simulink model "c166_user_io"  (Simulink 6.0)
settings: Solver=ode45  StartTime=0.0  StopTime=100  FixedStep=0.01  RelTol=1e-3
PreLoadFcn:
  | RTWConfigurationCB('preloadfcn', bdroot);
  | 
  | 
  | 
  | 
  | c166useriodata
libraries: c166drivers x1
CloseFcn:
  | rtwprivate ssgencode ModelCloseRequest c166_user_io
settings Model: Creator=The MathWorks Inc.  LastModifiedBy=batserve  ExtModeAutoUpdateStatusClock=off  ProdHWDeviceType=Infineon C16x
settings DataIOCC: SaveFormat=Structure  SignalLoggingName=sigsOut
settings OptimizationCC: InlineParams=on  InlineInvariantSignals=off  ZeroExternalMemoryAtStartup=off  ZeroInternalMemoryAtStartup=off  InitFltsAndDblsToZero=off  LifeSpan=1
settings DebuggingCC: CheckExecutionContextPreStartOutputMsg=on  CheckExecutionContextRuntimeOutputMsg=on  SolverPrmCheckMsg=none
settings HardwareCC: ProdBitPerInt=16  ProdEndianess=LittleEndian  ProdWordSize=16  ProdHWDeviceType=Infineon C16x  TargetHWDeviceType=32-bit Generic
settings RTWCC: SystemTargetFile=c166.tlc  MakeCommand=make_rtw_user  TemplateMakefile=c166.tmf  ProcessScript=c166_make_rtw_hook
settings CodeAppCC: IgnoreCustomStorageClasses=off
settings STFCustomTargetCC: TargetFcnLib=ansi_tfl_tmw.mat  GenFloatMathFcnCalls=ANSI_C  GenerateSampleERTMain=on  IncludeMdlTerminateFcn=off  CombineOutputUpdateFcns=on  ERTCustomFileBanners=on  SupportNonFinite=off  SupportComplex=off  PurelyIntegerCode=on  SystemTargetFile=c166.tlc
settings ERTTargetCC: TargetFcnLib=ansi_tfl_tmw.mat  GenFloatMathFcnCalls=ANSI_C  GenerateSampleERTMain=on  IncludeMdlTerminateFcn=off  SupportNonFinite=off  SupportComplex=off  PurelyIntegerCode=on  SupportContinuousTime=on  SupportNonInlinedSFcns=on  RootIOFormat=Individual Arguments  ERTCustomFileTemplate=example_file_process.tlc  InitialValueSource=Model
settings CustomProperty: DataType=RTWOptions_EnumType__toolbox_rtw_targets_c166_c166_c166_BuildActionC166  Value=Download_and_run
settings EnumStrPairs: String=Run_with_simulator

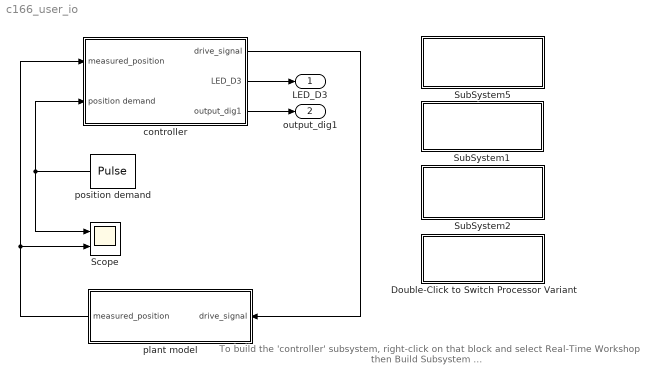
== system c166_user_io ==
  note: To build the 'controller'
      | subsystem, right-click
      | on that block and select
      | Real-Time Workshop
      | then Build Subsystem ...
  Double-Click to Switch Processor Variant : Subsystem  PropExecContextAcrossSSBoundary=on
      settings: OpenFcn=c166switchconfig(gcs)
      mask Display: disp('Switch Target\nProcessor Variant');
  Scope : Scope  NumInputPorts=2
      settings: YMin=0~0  YMax=600~600
  SubSystem1 : Subsystem  PropExecContextAcrossSSBoundary=on
      settings: OpenFcn=edit c166useriodata.m
      mask Display: disp('Open custom storage\nclass data file');
  SubSystem2 : Subsystem  PropExecContextAcrossSSBoundary=on
      settings: OpenFcn=helpview([docroot '/toolbox/c166/c166.map'], 'c166_user_io');
      mask Display: disp('Open help for\nintegrating hand code');
  SubSystem5 : Subsystem  PropExecContextAcrossSSBoundary=on
      settings: OpenFcn=|
      | edit([ matlabroot '/toolbox/rtw/targets/c166/c166demos/user_src/user_io.h'])
      | edit([ matlabroot '/toolbox/rtw/targets/c166/c166demos/user_src/user_io.c'])
      mask Display: disp('Open i/o driver\nsource files');
  controller : Subsystem  InitFcn=|  PropExecContextAcrossSSBoundary=on
      | % START RTW CONFIGURATION CODE %
      | RTWConfigurationCB('rtw_target_initfcn',gcb);
      | % END RTW CONFIGURATION CODE %
      mask Display: image(imread('target_affordance_icon.jpg'),'bottom-right')
  plant model : Subsystem  Orientation=left  PropExecContextAcrossSSBoundary=on
  position demand : DiscretePulseGenerator  Orientation=left  PulseType=Time based  Amplitude=uint16(512)  Period=5  PulseWidth=50
  LED_D3 : Outport
  output_dig1 : Outport  Port=2
  wires:
  controller/2(LED_D3) -> LED_D3/1
  controller/1(drive_signal) -> plant model/1(drive_signal)
  plant model/1(measured_position) -> controller/1(measured_position), Scope/2
  position demand/1 -> controller/2(position demand), Scope/1
  controller/3(output_dig1) -> output_dig1/1

== system c166_user_io/Double-Click to Switch Processor Variant ==

== system c166_user_io/SubSystem1 ==

== system c166_user_io/SubSystem2 ==

== system c166_user_io/SubSystem5 ==

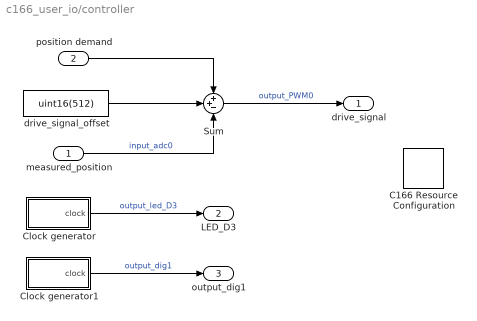
== system c166_user_io/controller ==
  measured_position : Inport  Port=1  SampleTime=0.001  LatchInput=off
  position demand : Inport  Port=2  SampleTime=0.001  LatchInput=off
  C166 Resource Configuration : c166drivers/C166 Resource Configuration  Tag=RTW CONFIGURATION BLOCK  Priority=-100000  oldParentName=c166_user_io/controller  oldBlockName=|  defaultConfigLibrary=c166drivers
      | c166_user_io/controller/C166
      | Resource
      | Configuration
  Clock generator : Subsystem  PropExecContextAcrossSSBoundary=on
  Clock generator1 : Subsystem  PropExecContextAcrossSSBoundary=on
  Sum : Sum  Inputs=++-  OutDataTypeMode=uint16  SaturateOnIntegerOverflow=on
  drive_signal_offset : Constant  Value=uint16(512)
  drive_signal : Outport
  LED_D3 : Outport  Port=2
  output_dig1 : Outport  Port=3
  wires:
  measured_position/1 -> Sum/3  "input_adc0"
  Sum/1 -> drive_signal/1  "output_PWM0"
  Clock generator/1(clock) -> LED_D3/1  "output_led_D3"
  drive_signal_offset/1 -> Sum/2
  position demand/1 -> Sum/1
  Clock generator1/1(clock) -> output_dig1/1  "output_dig1"

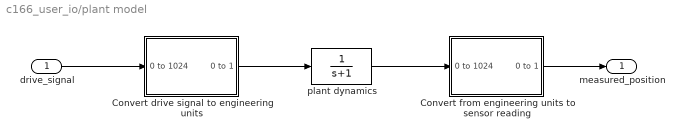
== system c166_user_io/plant model ==
  drive_signal : Inport  Port=1  LatchInput=off
  Convert drive signal to engineering units : Subsystem  PropExecContextAcrossSSBoundary=on
  Convert from engineering units to sensor reading : Subsystem  PropExecContextAcrossSSBoundary=on
  plant dynamics : TransferFcn  Denominator=[1 1]
  measured_position : Outport
  wires:
  drive_signal/1 -> Convert drive signal to engineering units/1(0 to 1024)
  Convert drive signal to engineering units/1(0 to 1) -> plant dynamics/1
  plant dynamics/1 -> Convert from engineering units to sensor reading/1(0 to 1024)
  Convert from engineering units to sensor reading/1(0 to 1) -> measured_position/1

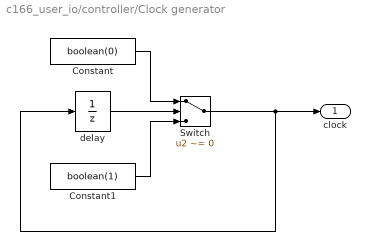
== system c166_user_io/controller/Clock generator ==
  Constant : Constant  Value=boolean(0)
  Constant1 : Constant  Value=boolean(1)
  Switch : Switch  Criteria=u2 ~= 0  SaturateOnIntegerOverflow=on
  delay : UnitDelay  X0=boolean(0)
  clock : Outport
  wires:
  delay/1 -> Switch/2
  Switch/1 -> clock/1, delay/1
  Constant/1 -> Switch/1
  Constant1/1 -> Switch/3

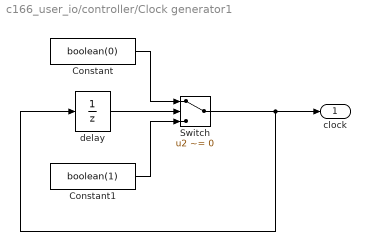
== system c166_user_io/controller/Clock generator1 ==
  Constant : Constant  Value=boolean(0)
  Constant1 : Constant  Value=boolean(1)
  Switch : Switch  Criteria=u2 ~= 0  SaturateOnIntegerOverflow=on
  delay : UnitDelay  X0=boolean(0)
  clock : Outport
  wires:
  Constant1/1 -> Switch/3
  Constant/1 -> Switch/1
  Switch/1 -> delay/1, clock/1
  delay/1 -> Switch/2

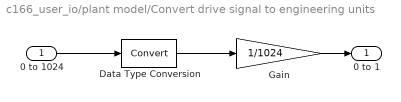
== system c166_user_io/plant model/Convert drive signal to engineering units ==
  0 to 1024 : Inport  Port=1  LatchInput=off
  Data Type Conversion : DataTypeConversion  OutDataTypeMode=double  SaturateOnIntegerOverflow=on  RndMeth=Zero
  Gain : Gain  Gain=1/1024  SaturateOnIntegerOverflow=on
  0 to 1 : Outport
  wires:
  Data Type Conversion/1 -> Gain/1
  0 to 1024/1 -> Data Type Conversion/1
  Gain/1 -> 0 to 1/1

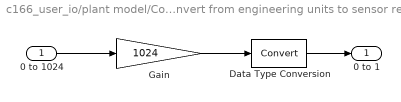
== system c166_user_io/plant model/Convert from engineering units to sensor reading ==
  0 to 1024 : Inport  Port=1  LatchInput=off
  Data Type Conversion : DataTypeConversion  OutDataTypeMode=uint16  SaturateOnIntegerOverflow=on  RndMeth=Zero
  Gain : Gain  Gain=1024  SaturateOnIntegerOverflow=on
  0 to 1 : Outport
  wires:
  0 to 1024/1 -> Gain/1
  Data Type Conversion/1 -> 0 to 1/1
  Gain/1 -> Data Type Conversion/1
